simulink library "m3_common_lib"  (R2021b)
settings: Solver=ode45  StartTime=0.0  StopTime=10.0  RelTol=1e-3
undefined symbols (not defined in the file or in its folder): ACCEL_PRE_MULT, APDT_SrvcMgr_IRVHVDCSubFcnReq, C_C1GearNumbers, C_C1GearRatios, C_Calibration, C_DitherWaveform, C_GearOffset, C_GearRatioIn, C_GearRatioInverseOut, C_GearRatioOut, CLUTCH_INNER_LOOP_UPDATE_RATE, CONSTANT, DEGRADED_MODE_SIZE, Dem_EventStatusType, DiscIntNeverNeededParam, F_FAULT_ENUM, F_NOFAULT, F_OUTOFRANGE, F_RATELIMIT, FALSE, FMI14_SPECIAL_INSTRUCTIONS, FMI20_DATA_DRIFTED_HIGH, FMI21_DATA_DRIFTED_LOW, FMI29_RESERVED_FOR_SAE_ASSIGNMENT, FMI30_RESERVED_FOR_SAE_ASSIGNMENT, FMI31_CONDITION_EXISTS, FMI32_NO_FAULT, IC, k_accel, k_mean, MAX_UINT32, MEAN_PRE_MULT, NTriggers, QLTY_SIGNAL_FAILED, QLTY_SIGNAL_FULLY_FUNCTION, QLTY_SIGNAL_SUBSTITUTED_BY_1ST_CHOICE, QLTY_SIGNAL_SUBSTITUTED_BY_2ND_CHOICE, QLTY_SIGNAL_SUBSTITUTED_BY_3RD_CHOICE, QLTY_SIGNAL_SUBSTITUTED_BY_4TH_CHOICE, SAMPLE_TIME_100us, simin, T_TestPoint, TF_FALSE, TF_TRUE, TimeStep, TRUE, WORKSPACE_UPDATE_RATE, Zero, ZERO
libraries: $bdroot x121, simulink x23, simulink_extras x4, MBD_EPS_Local_Blockset x4
(part 5 of 10)

== system m3_common_lib/Diag/Fault Injection ==
  note: Common Library::Diagnostics::Fault Injection
  input : Inport
  gain : Inport  Port=2
  offset : Inport  Port=3
  ulim : Inport  Port=4
  llim : Inport  Port=5
  hold : Inport  Port=6
  fl_trigger : Inport  Port=7
  Gain and Offset (in) : $bdroot/SCond/Gain and Offset (in)  DataType=Double
  OOR Fault Detection : $bdroot/Diag/OOR Fault Detection  InitialValue=InitialValue
  Switch : Switch  Threshold=0.5  ZeroCross=off
  Unit Delay : UnitDelay  InitialCondition=InitialValue  SampleTime=-1  HasFrameUpgradeWarning=on
  output : Outport  VectorParamsAs1DForOutWhenUnconnected=off
  hwfl : Outport  Port=2  VectorParamsAs1DForOutWhenUnconnected=off
  wires:
  Gain and Offset (in)/1 -> Switch/3
  Switch/1 -> OOR Fault Detection/1
  Unit Delay/1 -> Switch/1
  hold/1 -> Switch/2
  llim/1 -> OOR Fault Detection/3
  ulim/1 -> OOR Fault Detection/2
  fl_trigger/1 -> OOR Fault Detection/4
  OOR Fault Detection/2 -> hwfl/1
  OOR Fault Detection/1 -> Unit Delay/1, output/1
  offset/1 -> Gain and Offset (in)/3
  gain/1 -> Gain and Offset (in)/2
  input/1 -> Gain and Offset (in)/1

== system m3_common_lib/Diag/Fault Log ==
  note: Common Library::Diagnostics::Fault Log
  HWfl_Active : Inport  OutDataTypeStr=boolean
  HWfl_Events : Inport  Port=2  OutDataTypeStr=uint16
  HWfl_Frames : Inport  Port=3  OutDataTypeStr=uint32
  hold : Inport  Port=4  OutDataTypeStr=boolean
  Constant1 : Constant  Value=EVENT_ZERO
  Constant18 : Constant  Value=EVENT_MAX
  Constant2 : Constant  Value=EVENT_ONE
  Constant3 : Constant  Value=FRAME_ZERO
  Constant4 : Constant  Value=FRAME_MAX
  Constant5 : Constant  Value=FRAME_ONE
  Logical Operator1 : Logic
  Logical Operator3 : Logic
  Logical Operator8 : Logic
  Sat : $bdroot/Slink/Sat
  Sat1 : $bdroot/Slink/Sat
  Sum : Sum  Inputs=|++  InputSameDT=on  OutDataTypeStr=Inherit: Same as first input
  Sum1 : Sum  Inputs=|++  InputSameDT=on  OutDataTypeStr=Inherit: Same as first input
  Unit Delay1 : UnitDelay  InitialCondition=false  SampleTime=-1  HasFrameUpgradeWarning=on
  not1 : Logic  Operator=NOT
  not2 : Logic  Operator=NOT
  reset switch : Switch  Criteria=u2 ~= 0  Threshold=0.5  ZeroCross=off  InputSameDT=on
  reset switch1 : Switch  Criteria=u2 ~= 0  Threshold=0.5  ZeroCross=off  InputSameDT=on
  events : Outport  VectorParamsAs1DForOutWhenUnconnected=off
  frames : Outport  Port=2  VectorParamsAs1DForOutWhenUnconnected=off
  wires:
  Logical Operator3/1 -> reset switch/2
  Logical Operator8/1 -> not1/1, Logical Operator3/1
  Unit Delay1/1 -> Logical Operator3/2
  not1/1 -> Unit Delay1/1
  Logical Operator1/1 -> reset switch1/2
  hold/1 -> not2/1
  not2/1 -> Logical Operator8/2, Logical Operator1/1
  HWfl_Frames/1 -> Sum1/2, reset switch1/3
  HWfl_Events/1 -> Sum/2, reset switch/3
  Constant5/1 -> Sum1/1
  Sat1/1 -> frames/1
  Sum1/1 -> reset switch1/1
  reset switch1/1 -> Sat1/1
  Constant3/1 -> Sat1/3
  Constant4/1 -> Sat1/2
  Constant2/1 -> Sum/1
  Sat/1 -> events/1
  Sum/1 -> reset switch/1
  reset switch/1 -> Sat/1
  Constant1/1 -> Sat/3
  Constant18/1 -> Sat/2
  HWfl_Active/1 -> Logical Operator1/2, Logical Operator8/1

== system m3_common_lib/Diag/Fault_Cntr ==
  note: Common Library::Diagnostics::Fault Counter
  fl : Inport  OutDataTypeStr=boolean
  reset : Inport  Port=2  OutDataTypeStr=boolean
  fmi : Inport  Port=3  OutDataTypeStr=uint16
  Constant1 : Constant  Value=up_cnt
  Constant10 : Constant  Value=red_light  OutDataTypeStr=boolean
  Constant2 : Constant  Value=dn_cnt
  Constant3 : Constant  Value=fc_level  OutDataTypeStr=int16
  Constant4 : Constant  Value=fault_id  OutDataTypeStr=uint16
  Constant6 : Constant  Value=amber_light  OutDataTypeStr=boolean
  Data Type Conversion : DataTypeConversion  OutDataTypeStr=uint16
  Data Type Conversion1 : DataTypeConversion  OutDataTypeStr=boolean
  Data Type Conversion2 : DataTypeConversion  OutDataTypeStr=int16
  Data Type Conversion3 : DataTypeConversion  OutDataTypeStr=int16
  FaultHandlerCoreLogic : Subsystem  TreatAsAtomicUnit=on  RTWFcnName=FC_FMI_Handler
      settings: RTWFcnNameOpts=User specified  RTWFileNameOpts=Use function name
  Signal Conversion : SignalConversion  ConversionOutput=Contiguous copy  OverrideOpt=on
  Signal Conversion1 : SignalConversion  ConversionOutput=Contiguous copy  OverrideOpt=on
  inc switch : Switch  Criteria=u2 ~= 0  Threshold=0.5  ZeroCross=off  InputSameDT=on
  fc : Outport  OutDataTypeStr=uint16  VectorParamsAs1DForOutWhenUnconnected=off
  lights : Outport  Port=2  OutDataTypeStr=uint8  VectorParamsAs1DForOutWhenUnconnected=off
  wires:
  fl/1 -> inc switch/2
  reset/1 -> Data Type Conversion1/1
  FaultHandlerCoreLogic/1(fc) -> Signal Conversion/1
  fmi/1 -> Data Type Conversion/1
  FaultHandlerCoreLogic/2(lights) -> Signal Conversion1/1
  Signal Conversion/1 -> fc/1
  Signal Conversion1/1 -> lights/1
  Data Type Conversion/1 -> FaultHandlerCoreLogic/3(fmi)
  Data Type Conversion1/1 -> FaultHandlerCoreLogic/2(reset)
  Constant2/1 -> inc switch/3
  Constant3/1 -> Data Type Conversion3/1
  Constant4/1 -> FaultHandlerCoreLogic/5(fid)
  Constant10/1 -> FaultHandlerCoreLogic/6(red)
  Constant6/1 -> FaultHandlerCoreLogic/7(amber)
  Constant1/1 -> inc switch/1
  inc switch/1 -> Data Type Conversion2/1
  Data Type Conversion2/1 -> FaultHandlerCoreLogic/1(fl)
  Data Type Conversion3/1 -> FaultHandlerCoreLogic/4(fc_level)

== system m3_common_lib/Diag/Filter w Fault Handler ==
  input : Inport
  tau : Inport  Port=2
  override_value : Inport  Port=3
  override? : Inport  Port=4
  reset? : Inport  Port=5
  default : Inport  Port=6
  ramp_time : Inport  Port=7
  fault? : Inport  Port=8
  Data Type Conversion{,1..4} (5 alike) : DataTypeConversion  OutDataTypeStr=single
  Data Type Conversion5 : DataTypeConversion  OutDataTypeStr=boolean
  Data Type Conversion6 : DataTypeConversion  OutDataTypeStr=boolean
  Data Type Conversion7 : DataTypeConversion  OutDataTypeStr=boolean
  FilterWithFaultHandlerCoreLogic : Subsystem  TreatAsAtomicUnit=on  RTWFcnName=FLTRWROFH
      settings: RTWFcnNameOpts=User specified  RTWFileNameOpts=Use function name
  Signal Conversion : SignalConversion  ConversionOutput=Contiguous copy  OverrideOpt=on
  output : Outport  VectorParamsAs1DForOutWhenUnconnected=off
  wires:
  input/1 -> Data Type Conversion/1
  tau/1 -> Data Type Conversion1/1
  override_value/1 -> Data Type Conversion2/1
  FilterWithFaultHandlerCoreLogic/1(output) -> Signal Conversion/1
  override?/1 -> Data Type Conversion7/1
  reset?/1 -> Data Type Conversion6/1
  default/1 -> Data Type Conversion3/1
  ramp_time/1 -> Data Type Conversion4/1
  fault?/1 -> Data Type Conversion5/1
  Signal Conversion/1 -> output/1
  Data Type Conversion/1 -> FilterWithFaultHandlerCoreLogic/1(input)
  Data Type Conversion1/1 -> FilterWithFaultHandlerCoreLogic/2(tau)
  Data Type Conversion2/1 -> FilterWithFaultHandlerCoreLogic/3(override_value)
  Data Type Conversion3/1 -> FilterWithFaultHandlerCoreLogic/6(default)
  Data Type Conversion4/1 -> FilterWithFaultHandlerCoreLogic/7(ramp_time)
  Data Type Conversion5/1 -> FilterWithFaultHandlerCoreLogic/8(fault?)
  Data Type Conversion6/1 -> FilterWithFaultHandlerCoreLogic/5(reset?)
  Data Type Conversion7/1 -> FilterWithFaultHandlerCoreLogic/4(override?)

== system m3_common_lib/Diag/Filter w Fault Handler1 ==
  note: Common Library::Diagnostics::Filter With Fault Handler
  input : Inport
  tau : Inport  Port=2
  reset? : Inport  Port=3
  default : Inport  Port=4
  ramp_time : Inport  Port=5
  fault? : Inport  Port=6
  Abs1 : Abs  ZeroCross=off
  Abs2 : Abs  ZeroCross=off
  Constant5 : Constant  Value=TimeStep
  Fltr_wRO : Subsystem  RTWFcnName=FLTRWRO  mask(CL Filter wRO){TimeStep=TimeStep}
      mask prompts: TimeStep "Time Step"
      mask help:
      | First Order Filter, y(n)= T/tau x(n) + (1 - T/tau) y(n-1)
      |
      | If override is true (1) then output=override_value
      | If      reset is true (1) then output=input
      |    otherwise output = previous output + (input - previous output) * T/tau
      |
      | X(1) = input
      | X(2) = tau
      | X(3) = override value
      | X(4) = override flag
      | X(5) = reset flag
      |
      | Y(1) = output
      |
      | Time step is entered via mask parameter.
      | NgEK, Inc.
      mask init:
      | switch class(TimeStep)
      |  case ('double')
      |       IC = double(0.0);
      |     case ('single')
      |        IC = single(0.0);
      |     case ('int8')
      |          IC = int8(0);
      |     case ('int16')
      |       IC = int16(0);
      |    case ('int32')
      |         IC = int32(0);
      | end;
      settings: RTWFileNameOpts=Use function name
      mask Help: web(which(['common_lib17.html']))
      mask Display:
      | patch([0.4 0.4 0.6 0.6], [0.35 0.65 0.65 0.35], [255/255 127/255 255/255])
      | disp('Filter\nw RO')
      | port_label('input', 1, 'input')
      | port_label('input', 2, 'tau')
      | port_label('input', 3, 'override_value')
      | port_label('input', 4, 'override?')
      | port_label('input', 5, 'reset?')
      | port_label('output', 1, 'output')
  Product1 : Product  Inputs=**/  InputSameDT=on  OutDataTypeStr=Inherit: Same as first input
  Sum1 : Sum  Inputs=+-|  InputSameDT=on  OutDataTypeStr=Inherit: Same as first input
  Sum2 : Sum  Inputs=+-|  InputSameDT=on  OutDataTypeStr=Inherit: Same as first input
  Sum3 : Sum  Inputs=+-|  InputSameDT=on  OutDataTypeStr=Inherit: Same as first input
  Switch{1..4} (4 alike) : Switch  Threshold=0.5  ZeroCross=off  InputSameDT=on
  delay : UnitDelay  InitialCondition=Zero  SampleTime=-1  HasFrameUpgradeWarning=on
  ic: signal at fault : UnitDelay  InitialCondition=Zero  SampleTime=-1  HasFrameUpgradeWarning=on
  within zero tol of corrections : RelationalOperator  Operator=<  ZeroCross=off  RndMeth=Nearest
  output : Outport  VectorParamsAs1DForOutWhenUnconnected=off
  wires:
  Sum3/1 -> Abs1/1
  delay/1 -> Switch2/1
  Switch3/1 -> delay/1
  within zero tol of corrections/1 -> Switch3/2
  Abs2/1 -> within zero tol of corrections/1
  Abs1/1 -> within zero tol of corrections/2
  Sum2/1 -> Switch3/1
  Switch1/1 -> Sum3/1, Sum2/1
  Switch4/1 -> Switch1/3, Sum1/1, ic: signal at fault/1
  ic: signal at fault/1 -> Switch4/1
  Product1/1 -> Abs2/1, Sum2/2
  Constant5/1 -> Product1/2
  Sum1/1 -> Product1/1
  default/1 -> Sum3/2, Switch3/3, Sum1/2
  Fltr_wRO/1(output) -> Switch4/3, output/1
  input/1 -> Switch2/3
  Switch2/1 -> Switch1/1, Fltr_wRO/1(input)
  reset?/1 -> Fltr_wRO/3(reset?)
  tau/1 -> Fltr_wRO/2(tau)
  fault?/1 -> Switch1/2, Switch4/2, Switch2/2
  ramp_time/1 -> Product1/3

== system m3_common_lib/Diag/OOR Fault Detection ==
  note: Common Library::Diagnostics::Out of Range Fault Detection
  in : Inport
  ulim : Inport  Port=2
  llim : Inport  Port=3
  ext_fault? : Inport  Port=4
  Logical Operator : Logic  Operator=OR  Inputs=3  AllPortsSameDT=off
  Relational Operator : RelationalOperator  Operator=<  ZeroCross=off  RndMeth=Nearest
  Relational Operator1 : RelationalOperator  Operator=<  ZeroCross=off  RndMeth=Nearest
  Sat : $bdroot/Slink/Sat
  Switch : Switch  Threshold=0.5  ZeroCross=off
  Unit Delay : UnitDelay  InitialCondition=InitialValue  SampleTime=-1  HasFrameUpgradeWarning=on
  out : Outport  VectorParamsAs1DForOutWhenUnconnected=off
  fault? : Outport  Port=2  VectorParamsAs1DForOutWhenUnconnected=off
  wires:
  Sat/1 -> Unit Delay/1, out/1
  Switch/1 -> Sat/1
  ext_fault?/1 -> Logical Operator/3
  llim/1 -> Sat/3, Relational Operator/2
  ulim/1 -> Relational Operator1/1, Sat/2
  in/1 -> Relational Operator1/2, Relational Operator/1, Switch/3
  Relational Operator1/1 -> Logical Operator/1
  Relational Operator/1 -> Logical Operator/2
  Logical Operator/1 -> Switch/2, fault?/1
  Unit Delay/1 -> Switch/1

== system m3_common_lib/Diag/Rate Limit Fault Detection ==
  note: Common Library::Diagnostics::Rate Limit Fault Detection
  in : Inport
  rlim : Inport  Port=2
  ext_fault? : Inport  Port=3
  Constant1 : Constant  Value=true
  Constant2 : Constant  Value=TimeStep
  Data Type Conversion : DataTypeConversion  OutDataTypeStr=single
  OOR Fault Detection : $bdroot/Diag/OOR Fault Detection  InitialValue=IC
  Product1 : Product  InputSameDT=on  OutDataTypeStr=Inherit: Same as first input
  Sum1 : Sum  Inputs=-+|  InputSameDT=on  OutDataTypeStr=Inherit: Same as first input
  Sum2 : Sum  Inputs=|++  InputSameDT=on  OutDataTypeStr=Inherit: Same as first input
  Sum3 : Sum  Inputs=++|  InputSameDT=on  OutDataTypeStr=Inherit: Same as first input
  Unit Delay : UnitDelay  InitialCondition=Zero  SampleTime=-1  HasFrameUpgradeWarning=on
      settings: AttributesFormatString=ic=%<X0>
  Unit Delay1 : UnitDelay  InitialCondition=false  SampleTime=-1  HasFrameUpgradeWarning=on
      settings: AttributesFormatString=ic=%<X0>
  Unit Delay2 : UnitDelay  InitialCondition=Zero  SampleTime=-1  HasFrameUpgradeWarning=on
      settings: AttributesFormatString=ic=%<X0>
  Unit Delay3 : UnitDelay  InitialCondition=false  SampleTime=-1  HasFrameUpgradeWarning=on
      settings: AttributesFormatString=ic=%<X0>
  inc switch : Switch  Threshold=0.5  ZeroCross=off  InputSameDT=on
  inc switch1 : Switch  Threshold=0.5  ZeroCross=off  InputSameDT=on
  out : Outport  VectorParamsAs1DForOutWhenUnconnected=off
  fault? : Outport  Port=2  VectorParamsAs1DForOutWhenUnconnected=off
  wires:
  Constant2/1 -> Data Type Conversion/1
  Data Type Conversion/1 -> Product1/1
  inc switch1/1 -> Sum2/1, Sum1/2
  Unit Delay3/1 -> inc switch1/2
  Constant1/1 -> Unit Delay3/1
  Unit Delay/1 -> inc switch1/1
  Unit Delay1/1 -> inc switch/2
  Unit Delay2/1 -> Sum3/1
  Sum3/1 -> inc switch/1
  Product1/1 -> Sum3/2, inc switch/3
  rlim/1 -> Product1/2
  inc switch/1 -> Unit Delay2/1, Sum1/1, Sum2/2
  Sum2/1 -> OOR Fault Detection/2
  Sum1/1 -> OOR Fault Detection/3
  OOR Fault Detection/2 -> Unit Delay1/1, fault?/1
  OOR Fault Detection/1 -> Unit Delay/1, out/1
  ext_fault?/1 -> OOR Fault Detection/4
  in/1 -> inc switch1/3, OOR Fault Detection/1

== system m3_common_lib/Diagnostics/Calibration Enabled Debounce ==
  diagInput : Inport
  diagStartUpComp : Inport  Port=2
  diagMaxVal : Inport  Port=3
  diagMinVal : Inport  Port=4
  diagUpCnt : Inport  Port=5
  diagDnCnt : Inport  Port=6
  diagFaultCntThresh : Inport  Port=7
  diagPassCntThresh : Inport  Port=8
  diagDbncEnab : Inport  Port=9
  diagReset : Inport  Port=10
  diagEnable : Inport  Port=11
  diagHealEn : Inport  Port=12
  DiagFaultCounter : $bdroot/Diagnostics/DiagFaultCounter  SystemSampleTime=-1  VariantActivationTime=update diagram  Latency=0  AutoFrameSizeCalculation=off
  OR : Logic  Operator=OR  AllPortsSameDT=off  OutDataTypeStr=boolean
  Relational Operator : RelationalOperator  OutDataTypeStr=boolean  ZeroCross=off  RndMeth=Nearest
  Relational Operator1 : RelationalOperator  Operator=<=  OutDataTypeStr=boolean  ZeroCross=off  RndMeth=Nearest
  diagFaultStatus : Outport  OutputWhenDisabled=reset  InitialOutput=Dem_EventStatusType.DEM_EVENT_STATUS_INIT  VectorParamsAs1DForOutWhenUnconnected=off
  wires:
  diagHealEn/1 -> DiagFaultCounter/10
  diagPassCntThresh/1 -> DiagFaultCounter/7
  diagMaxVal/1 -> Relational Operator/2
  diagMinVal/1 -> Relational Operator1/2
  Relational Operator/1 -> OR/1
  Relational Operator1/1 -> OR/2
  diagInput/1 -> Relational Operator/1, Relational Operator1/1
  OR/1 -> DiagFaultCounter/1
  diagStartUpComp/1 -> DiagFaultCounter/2
  diagReset/1 -> DiagFaultCounter/3
  diagEnable/1 -> DiagFaultCounter/4
  diagDbncEnab/1 -> DiagFaultCounter/5
  diagFaultCntThresh/1 -> DiagFaultCounter/6
  diagUpCnt/1 -> DiagFaultCounter/8
  diagDnCnt/1 -> DiagFaultCounter/9
  DiagFaultCounter/1 -> diagFaultStatus/1

== system m3_common_lib/Diagnostics/Calibration Enabled Debounce Boolean Input ==
  diagInput : Inport
  diagStartUpComp : Inport  Port=2
  diagUpCnt : Inport  Port=3
  diagDnCnt : Inport  Port=4
  diagFaultCntThresh : Inport  Port=5
  diagPassCntThresh : Inport  Port=6
  diagDbncEnab : Inport  Port=7
  diagReset : Inport  Port=8
  diagEnable : Inport  Port=9
  diagHealEn : Inport  Port=10
  DiagFaultCounter : $bdroot/Diagnostics/DiagFaultCounter  SystemSampleTime=-1  VariantActivationTime=update diagram  Latency=0  AutoFrameSizeCalculation=off
  diagFaultStatus : Outport  OutputWhenDisabled=reset  InitialOutput=Dem_EventStatusType.DEM_EVENT_STATUS_INIT  VectorParamsAs1DForOutWhenUnconnected=off
  wires:
  DiagFaultCounter/1 -> diagFaultStatus/1
  diagDnCnt/1 -> DiagFaultCounter/9
  diagUpCnt/1 -> DiagFaultCounter/8
  diagFaultCntThresh/1 -> DiagFaultCounter/6
  diagDbncEnab/1 -> DiagFaultCounter/5
  diagEnable/1 -> DiagFaultCounter/4
  diagReset/1 -> DiagFaultCounter/3
  diagStartUpComp/1 -> DiagFaultCounter/2
  diagInput/1 -> DiagFaultCounter/1
  diagPassCntThresh/1 -> DiagFaultCounter/7
  diagHealEn/1 -> DiagFaultCounter/10

== system m3_common_lib/Diagnostics/Calibration Enabled MinMax OOR ==
  Input : Inport
  ULim : Inport  Port=2
  LLim : Inport  Port=3
  Cal_Enable : Inport  Port=4
  Ext_Fault : Inport  Port=5
  Enabled OOR : Subsystem  mask(Enabled OOR Subsystem){InitialValue=InitialValue, InDataType=single}
      mask prompts: InitialValue "Initial Value"; InDataType "Input Data Type"
      mask init:
      | DataType = get_param(gcb, 'InDataType');
      | Capture1 = [gcb '/OOR MinMax Capture/CL MinMax Capture'];
      | Capture2 = [gcb '/OOR MinMax Capture/CL MinMax Capture1'];
      | 
      | set_param(Capture1, 'InDataType', DataType);
      | set_param(Capture2, 'InDataType', DataType);
      mask TypeOptions InDataType: single | int16
  Switch : Switch  Threshold=0.5  ZeroCross=off
  Switch1 : Switch  Threshold=0.5  ZeroCross=off
  Out : Outport  VectorParamsAs1DForOutWhenUnconnected=off
  Max_Value : Outport  Port=2  VectorParamsAs1DForOutWhenUnconnected=off
  Min_Value : Outport  Port=3  VectorParamsAs1DForOutWhenUnconnected=off
  Fault : Outport  Port=4  VectorParamsAs1DForOutWhenUnconnected=off
  wires:
  Input/1 -> Enabled OOR/1(In), Switch/3
  ULim/1 -> Enabled OOR/2(ULim)
  LLim/1 -> Enabled OOR/3(LLim)
  Ext_Fault/1 -> Enabled OOR/4(Ext_Fault), Switch1/3
  Switch/1 -> Out/1
  Switch1/1 -> Fault/1
  Enabled OOR/1(Out) -> Switch/1
  Cal_Enable/1 -> Switch1/2, Switch/2, Enabled OOR/Enable
  Enabled OOR/2(Fault) -> Switch1/1
  Enabled OOR/3(Max) -> Max_Value/1
  Enabled OOR/4(Min) -> Min_Value/1

== system m3_common_lib/Diagnostics/Calibration Enabled MinMax RLim ==
  Input : Inport
  Rate_Limit : Inport  Port=2
  Cal_Enable : Inport  Port=3
  Ext_Fault : Inport  Port=4
  Enabled RLim : Subsystem  mask(Enablede Rate Limit Fault Detection){IC=IC, TimeStep=TimeStep, InDataType=single}
      mask prompts: IC "Initial Condition"; TimeStep "Update Time"; InDataType "Input Data Type"
      mask init:
      | DataType = get_param(gcb, 'InDataType');
      | Capture1 = [gcb '/RLim MinMax Capture/CL MinMax Capture'];
      | Capture2 = [gcb '/RLim MinMax Capture/CL MinMax Capture1'];
      | 
      | set_param(Capture1, 'InDataType', DataType);
      | set_param(Capture2, 'InDataType', DataType);
      mask TypeOptions InDataType: single | int16
  Switch : Switch  Threshold=0.5  ZeroCross=off
  Switch1 : Switch  Threshold=0.5  ZeroCross=off
  Out : Outport  VectorParamsAs1DForOutWhenUnconnected=off
  Max Pos Rate : Outport  Port=2  VectorParamsAs1DForOutWhenUnconnected=off
  Max Neg Rate : Outport  Port=3  VectorParamsAs1DForOutWhenUnconnected=off
  Fault : Outport  Port=4  VectorParamsAs1DForOutWhenUnconnected=off
  wires:
  Cal_Enable/1 -> Switch/2, Switch1/2, Enabled RLim/Enable
  Input/1 -> Switch/3, Enabled RLim/1(In)
  Switch/1 -> Out/1
  Switch1/1 -> Fault/1
  Rate_Limit/1 -> Enabled RLim/2(RLim)
  Enabled RLim/1(out) -> Switch/1
  Enabled RLim/2(fault?) -> Switch1/1
  Ext_Fault/1 -> Enabled RLim/3(Ext_Fault), Switch1/3
  Enabled RLim/3(Max Pos Rate) -> Max Pos Rate/1
  Enabled RLim/4(Max Neg Rate) -> Max Neg Rate/1

== system m3_common_lib/Diagnostics/Ccaller_DiagLv1 ==
  diagFaultActive : Inport
  diagStartUpComp : Inport  Port=2
  diagReset : Inport  Port=3
  diagEnable : Inport  Port=4
  diagDbncEnable : Inport  Port=5
  diagFaultCntThresh : Inport  Port=6
  diagPassCntThresh : Inport  Port=7
  diagUpCnt : Inport  Port=8
  diagDnCnt : Inport  Port=9
  diagHealEn : Inport  Port=10
  diagPrestorageEn : Inport  Port=11
  diagJumpDownEn : Inport  Port=12
  DiagDebounceLv1_CCaller : CCaller  FunctionName=DiagDebounceLv1  PortSpecificationStruct="%)30     .    <!<   8    (     @         %    \"     T    !     0         %  0 \"0    $    _    07)G3F%M90  4&]R=$YA;64 4V-O<&4     26YD97@     5'EP90      4VEZ90      27-';&]B86P   X   !     !@    @    $          4    (     0   !     !         !     0    9&EA9T9A=6QT0V]U;G1E<@X   !     !@    @    $          4    (     0   !     !         !     0    9&EA9T9A=6QT0V]U;G1E<@X   !     !@    @    $     ...(+7711 chars)"
  Unit Delay : UnitDelay  InitialCondition=int16(0)  SampleTime=-1  HasFrameUpgradeWarning=on
      settings: AttributesFormatString=%<InitialCondition>
  Unit Delay1 : UnitDelay  InitialCondition=uint8(32)  SampleTime=-1  HasFrameUpgradeWarning=on
      settings: AttributesFormatString=%<InitialCondition>
  Unit Delay2 : UnitDelay  InitialCondition=false  SampleTime=-1  HasFrameUpgradeWarning=on
      settings: AttributesFormatString=%<InitialCondition>
  Unit Delay3 : UnitDelay  InitialCondition=false  SampleTime=-1  HasFrameUpgradeWarning=on
      settings: AttributesFormatString=%<InitialCondition>
  Unit Delay4 : UnitDelay  InitialCondition=false  SampleTime=-1  HasFrameUpgradeWarning=on
      settings: AttributesFormatString=%<InitialCondition>
  diagFaultStatus : Outport  VectorParamsAs1DForOutWhenUnconnected=off
  diagPrestorageTrigger : Outport  Port=2  VectorParamsAs1DForOutWhenUnconnected=off
  wires:
  diagJumpDownEn/1 -> ?
  Unit Delay4/1 -> DiagDebounceLv1_CCaller/4
  ? -> Unit Delay4/1
  diagPrestorageEn/1 -> ?
  Unit Delay3/1 -> DiagDebounceLv1_CCaller/5
  ? -> diagPrestorageTrigger/1, Unit Delay3/1
  Unit Delay2/1 -> DiagDebounceLv1_CCaller/3
  DiagDebounceLv1_CCaller/3 -> Unit Delay2/1
  Unit Delay1/1 -> DiagDebounceLv1_CCaller/2
  DiagDebounceLv1_CCaller/2 -> Unit Delay1/1, diagFaultStatus/1
  Unit Delay/1 -> DiagDebounceLv1_CCaller/1
  DiagDebounceLv1_CCaller/1 -> Unit Delay/1
  diagPassCntThresh/1 -> DiagDebounceLv1_CCaller/12
  diagDbncEnable/1 -> DiagDebounceLv1_CCaller/10
  diagEnable/1 -> DiagDebounceLv1_CCaller/9
  diagHealEn/1 -> ?
  diagFaultActive/1 -> DiagDebounceLv1_CCaller/6
  diagFaultCntThresh/1 -> DiagDebounceLv1_CCaller/11
  diagReset/1 -> DiagDebounceLv1_CCaller/8
  diagDnCnt/1 -> ?
  diagStartUpComp/1 -> DiagDebounceLv1_CCaller/7
  diagUpCnt/1 -> DiagDebounceLv1_CCaller/13

== system m3_common_lib/Diagnostics/Ccaller_DiagLv2 ==
  diagFaultActive : Inport
  diagStartUpComp : Inport  Port=2
  diagReset : Inport  Port=3
  diagFaultCntThresh : Inport  Port=4
  diagUpCnt : Inport  Port=5
  diagDnCnt : Inport  Port=6
  diagHealEn : Inport  Port=7
  DiagDebounceLv2_CCaller : CCaller  FunctionName=DiagDebounceLv2  PortSpecificationStruct="%)30     .    8!$   8    (     @         %    \"     L    !     0         %  0 \"0    $    V    07)G3F%M90  4&]R=$YA;64 4V-O<&4     26YD97@     5'EP90      4VEZ90         .    ,     8    (    !          %    \"     $    #     0         0  , ;W5T  X    P    !@    @    $          4    (     0    ,    !         !   P!O=70 #@   #@    &    \"     0         !0    @    !    !@    $         $     8   !/=7 ...(+5614 chars)"
  Unit Delay : UnitDelay  InitialCondition=int16(0)  SampleTime=-1  HasFrameUpgradeWarning=on
      settings: AttributesFormatString=%<InitialCondition>
  Unit Delay1 : UnitDelay  InitialCondition=uint8(0)  SampleTime=-1  HasFrameUpgradeWarning=on
      settings: AttributesFormatString=%<InitialCondition>
  Unit Delay2 : UnitDelay  InitialCondition=int16(0)  SampleTime=-1  HasFrameUpgradeWarning=on
      settings: AttributesFormatString=%<InitialCondition>
  diagFaultStatus : Outport  VectorParamsAs1DForOutWhenUnconnected=off
  wires:
  diagUpCnt/1 -> DiagDebounceLv2_CCaller/8
  diagStartUpComp/1 -> DiagDebounceLv2_CCaller/5
  diagDnCnt/1 -> DiagDebounceLv2_CCaller/9
  diagReset/1 -> DiagDebounceLv2_CCaller/6
  DiagDebounceLv2_CCaller/1 -> diagFaultStatus/1
  diagFaultCntThresh/1 -> DiagDebounceLv2_CCaller/7
  diagFaultActive/1 -> DiagDebounceLv2_CCaller/4
  diagHealEn/1 -> DiagDebounceLv2_CCaller/10
  DiagDebounceLv2_CCaller/2 -> Unit Delay/1
  Unit Delay/1 -> DiagDebounceLv2_CCaller/1
  DiagDebounceLv2_CCaller/3 -> Unit Delay1/1
  Unit Delay1/1 -> DiagDebounceLv2_CCaller/2
  DiagDebounceLv2_CCaller/4 -> Unit Delay2/1
  Unit Delay2/1 -> DiagDebounceLv2_CCaller/3

== system m3_common_lib/Diagnostics/DiagFaultCounter ==
  diagFaultActive : Inport
  diagStartUpComp : Inport  Port=2
  diagReset : Inport  Port=3
  diagEnable : Inport  Port=4
  diagDbncEnab : Inport  Port=5
  diagFaultCntThresh : Inport  Port=6
  diagPassCntThresh : Inport  Port=7
  diagUpCnt : Inport  Port=8
  diagDnCnt : Inport  Port=9
  diagHealEn : Inport  Port=10
  DiagFaulCounter : Stateflow chart  TreatAsAtomicUnit=on
  diagFaultStatus : Outport  OutputWhenDisabled=reset  InitialOutput=Dem_EventStatusType.DEM_EVENT_STATUS_INIT  VectorParamsAs1DForOutWhenUnconnected=off
  wires:
  diagHealEn/1 -> DiagFaulCounter/10(diagHealEn)
  diagPassCntThresh/1 -> DiagFaulCounter/7(diagPassCntThresh)
  diagStartUpComp/1 -> DiagFaulCounter/2(diagStartUpComp)
  diagDbncEnab/1 -> DiagFaulCounter/5(diagDbncEnab)
  DiagFaulCounter/1(diagFaultStatus) -> diagFaultStatus/1
  diagEnable/1 -> DiagFaulCounter/4(diagEnable)
  diagDnCnt/1 -> DiagFaulCounter/9(diagDnCnt)
  diagUpCnt/1 -> DiagFaulCounter/8(diagUpCnt)
  diagReset/1 -> DiagFaulCounter/3(diagReset)
  diagFaultCntThresh/1 -> DiagFaulCounter/6(diagFaultCntThresh)
  diagFaultActive/1 -> DiagFaulCounter/1(diagFaultActive)

== system m3_common_lib/Diagnostics/ExtractValue ==
  in : Inport  OutDataTypeStr=Bus: BO_InputSignal
  Bus Selector : BusSelector  OutputSignals=value,FMI
  value : Outport  VectorParamsAs1DForOutWhenUnconnected=off
  FMI : Outport  Port=2  VectorParamsAs1DForOutWhenUnconnected=off
  wires:
  Bus Selector/2 -> FMI/1  "<FMI>"
  in/1 -> Bus Selector/1
  Bus Selector/1 -> value/1  "<value>"

== system m3_common_lib/Diagnostics/FMIUpdate ==
  UpdateFaultStatus : Inport
  FMI_In : Inport  Port=2
  FMI_UpdateValue : Inport  Port=3
  Constant2 : Constant  Value=FMI32_NO_FAULT  SampleTime=-1
  Relational Operator3 : RelationalOperator  Operator=~=  ZeroCross=off  RndMeth=Nearest
  Switch : Switch  Threshold=0.5  ZeroCross=off
  Switch1 : Switch  Threshold=0.5  ZeroCross=off
  FMI_Out : Outport  VectorParamsAs1DForOutWhenUnconnected=off
  wires:
  Switch1/1 -> FMI_Out/1
  FMI_In/1 -> Switch/3, Switch1/1, Relational Operator3/1
  Relational Operator3/1 -> Switch1/2
  Switch/1 -> Switch1/3
  FMI_UpdateValue/1 -> Switch/1
  UpdateFaultStatus/1 -> Switch/2
  Constant2/1 -> Relational Operator3/2

== system m3_common_lib/Diagnostics/Fault Debounce Lv1 Boolean Input ==
  diagInput : Inport
  diagStartUpComp : Inport  Port=2
  diagUpCnt : Inport  Port=3
  diagDnCnt : Inport  Port=4
  diagFaultCntThresh : Inport  Port=5
  diagPassCntThresh : Inport  Port=6
  diagDbncEnab : Inport  Port=7
  diagReset : Inport  Port=8
  diagEnable : Inport  Port=9
  diagHealEn : Inport  Port=10
  diagPreestorageEn : Inport  Port=11
  diagJumpDownEn : Inport  Port=12
  Ccaller_DiagLv1 : $bdroot/Diagnostics/Ccaller_DiagLv1  SystemSampleTime=-1  VariantActivationTime=update diagram  Latency=0  AutoFrameSizeCalculation=off
  diagFaultStatus : Outport  OutputWhenDisabled=reset  InitialOutput=Dem_EventStatusType.DEM_EVENT_STATUS_INIT  VectorParamsAs1DForOutWhenUnconnected=off
  diagPreestorageTrigger : Outport  Port=2  OutputWhenDisabled=reset  InitialOutput=Dem_EventStatusType.DEM_EVENT_STATUS_INIT  VectorParamsAs1DForOutWhenUnconnected=off
  wires:
  diagStartUpComp/1 -> Ccaller_DiagLv1/2
  diagReset/1 -> Ccaller_DiagLv1/3
  diagEnable/1 -> Ccaller_DiagLv1/4
  diagDbncEnab/1 -> Ccaller_DiagLv1/5
  diagFaultCntThresh/1 -> Ccaller_DiagLv1/6
  diagPassCntThresh/1 -> Ccaller_DiagLv1/7
  diagUpCnt/1 -> Ccaller_DiagLv1/8
  diagDnCnt/1 -> Ccaller_DiagLv1/9
  diagHealEn/1 -> Ccaller_DiagLv1/10
  diagPreestorageEn/1 -> Ccaller_DiagLv1/11
  diagJumpDownEn/1 -> Ccaller_DiagLv1/12
  Ccaller_DiagLv1/2 -> diagPreestorageTrigger/1
  Ccaller_DiagLv1/1 -> diagFaultStatus/1
  diagInput/1 -> Ccaller_DiagLv1/1

== system m3_common_lib/Diagnostics/Fault Debounce Lv1 state Input ==
  diagInput : Inport
  diagStartUpComp : Inport  Port=2
  diagMaxVal : Inport  Port=3
  diagMinVal : Inport  Port=4
  diagUpCnt : Inport  Port=5
  diagDnCnt : Inport  Port=6
  diagFaultCntThresh : Inport  Port=7
  diagPassCntThresh : Inport  Port=8
  diagDbncEnab : Inport  Port=9
  diagReset : Inport  Port=10
  diagEnable : Inport  Port=11
  diagHealEn : Inport  Port=12
  diagPreestorageEn : Inport  Port=13
  diagJumpDownEn : Inport  Port=14
  Ccaller_DiagLv1 : $bdroot/Diagnostics/Ccaller_DiagLv1  SystemSampleTime=-1  VariantActivationTime=update diagram  Latency=0  AutoFrameSizeCalculation=off
  OR : Logic  Operator=OR  AllPortsSameDT=off  OutDataTypeStr=boolean
  Relational Operator : RelationalOperator  OutDataTypeStr=boolean  ZeroCross=off  RndMeth=Nearest
  Relational Operator1 : RelationalOperator  Operator=<=  OutDataTypeStr=boolean  ZeroCross=off  RndMeth=Nearest
  diagFaultStatus : Outport  OutputWhenDisabled=reset  InitialOutput=Dem_EventStatusType.DEM_EVENT_STATUS_INIT  VectorParamsAs1DForOutWhenUnconnected=off
  diagPreestorageTrigger : Outport  Port=2  OutputWhenDisabled=reset  InitialOutput=Dem_EventStatusType.DEM_EVENT_STATUS_INIT  VectorParamsAs1DForOutWhenUnconnected=off
  wires:
  diagMaxVal/1 -> Relational Operator/2
  diagReset/1 -> Ccaller_DiagLv1/3
  diagDnCnt/1 -> Ccaller_DiagLv1/9
  diagFaultCntThresh/1 -> Ccaller_DiagLv1/6
  diagPassCntThresh/1 -> Ccaller_DiagLv1/7
  diagUpCnt/1 -> Ccaller_DiagLv1/8
  Relational Operator/1 -> OR/1
  diagStartUpComp/1 -> Ccaller_DiagLv1/2
  diagDbncEnab/1 -> Ccaller_DiagLv1/5
  diagInput/1 -> Relational Operator/1, Relational Operator1/1
  diagHealEn/1 -> Ccaller_DiagLv1/10
  diagMinVal/1 -> Relational Operator1/2
  OR/1 -> Ccaller_DiagLv1/1
  Relational Operator1/1 -> OR/2
  diagEnable/1 -> Ccaller_DiagLv1/4
  diagPreestorageEn/1 -> Ccaller_DiagLv1/11
  diagJumpDownEn/1 -> Ccaller_DiagLv1/12
  Ccaller_DiagLv1/1 -> diagFaultStatus/1
  Ccaller_DiagLv1/2 -> diagPreestorageTrigger/1

== system m3_common_lib/Diagnostics/FaultStatusUpdate ==
  FMI_In : Inport
  DriftLow : Inport  Port=2
  DriftHigh : Inport  Port=3
  SpecialInstructions : Inport  Port=4
  ConditionExists : Inport  Port=5
  DriftLowSubReqest : Inport  Port=6
  DriftLowSubReqest1 : Inport  Port=7
  Constant : Constant  Value=FMI14_SPECIAL_INSTRUCTIONS  SampleTime=-1
  Constant1 : Constant  Value=FMI21_DATA_DRIFTED_LOW  SampleTime=-1
  Constant2 : Constant  Value=FMI20_DATA_DRIFTED_HIGH  SampleTime=-1
  Constant3 : Constant  Value=FMI29_RESERVED_FOR_SAE_ASSIGNMENT  SampleTime=-1
  Constant4 : Constant  Value=FMI32_NO_FAULT  SampleTime=-1
  Constant5 : Constant  Value=FMI30_RESERVED_FOR_SAE_ASSIGNMENT  SampleTime=-1
  Constant6 : Constant  Value=FMI31_CONDITION_EXISTS  SampleTime=-1
  Relational Operator3 : RelationalOperator  Operator=~=  ZeroCross=off  RndMeth=Nearest
  Switch{,1..6} (7 alike) : Switch  Threshold=0.5  ZeroCross=off
  FMI_Out : Outport  VectorParamsAs1DForOutWhenUnconnected=off
  wires:
  Switch1/1 -> FMI_Out/1
  Constant4/1 -> Relational Operator3/2
  Switch/1 -> Switch1/3
  Relational Operator3/1 -> Switch1/2
  FMI_In/1 -> Relational Operator3/1, Switch1/1, Switch6/3
  Switch2/1 -> Switch/3
  Switch3/1 -> Switch2/3
  Switch4/1 -> Switch3/3
  DriftLow/1 -> Switch/2
  Constant1/1 -> Switch/1
  Constant2/1 -> Switch2/1
  DriftHigh/1 -> Switch2/2
  Constant/1 -> Switch3/1
  SpecialInstructions/1 -> Switch3/2
  Constant6/1 -> Switch4/1
  ConditionExists/1 -> Switch4/2
  Constant3/1 -> Switch5/1
  DriftLowSubReqest/1 -> Switch5/2
  Constant5/1 -> Switch6/1
  DriftLowSubReqest1/1 -> Switch6/2
  Switch6/1 -> Switch5/3
  Switch5/1 -> Switch4/3

== system m3_common_lib/Diagnostics/KeepAlive ==
  State : Inport  OutDataTypeStr=boolean  PortDimensions=1
  A : Inport  Port=2  PortDimensions=1
  B : Inport  Port=3  PortDimensions=1
  Delay : UnitDelay  InitialCondition=false  SampleTime=-1  HasFrameUpgradeWarning=on
  Logical Operator : Logic  Operator=OR  AllPortsSameDT=off  OutDataTypeStr=boolean
  RelOp : RelationalOperator  Operator===  OutDataTypeStr=boolean  RndMeth=Nearest  InputSameDT=on
  Enable : Outport  OutDataTypeStr=boolean  PortDimensions=1  VectorParamsAs1DForOutWhenUnconnected=off
  Rel : Outport  Port=2  OutDataTypeStr=boolean  PortDimensions=1  VectorParamsAs1DForOutWhenUnconnected=off
  wires:
  RelOp/1 -> Logical Operator/2, Rel/1
  Logical Operator/1 -> Enable/1
  B/1 -> RelOp/2
  Delay/1 -> Logical Operator/1
  State/1 -> Delay/1
  A/1 -> RelOp/1

== system m3_common_lib/Diagnostics/LogicBasedActivation ==
  note: Logic Based Activation
  Enable : Inport  OutDataTypeStr=boolean  PortDimensions=1
  DMToAdd : Inport  Port=2  OutDataTypeStr=uint32  PortDimensions=DM_SIZE
  Add : Inport  Port=3  OutDataTypeStr=boolean  PortDimensions=1
  DMPackedData_in : Inport  Port=4  OutDataTypeStr=uint32  PortDimensions=DM_SIZE
  Bitwise Operator : simulink/Logic and Bit Operations/Bitwise Operator  logicop=OR  UseBitMask=off  NumInputPorts=2  BitMask=bin2dec('11011001')  BitMaskRealWorld=Stored Integer
  Logical Operator1 : Logic  AllPortsSameDT=off
  Switch3 : Switch  Threshold=0.5  ZeroCross=off
  DMPackedData_out : Outport  OutDataTypeStr=uint32  PortDimensions=DM_SIZE  VectorParamsAs1DForOutWhenUnconnected=off
  wires:
  Switch3/1 -> DMPackedData_out/1
  Bitwise Operator/1 -> Switch3/1
  DMToAdd/1 -> Bitwise Operator/1
  DMPackedData_in/1 -> Bitwise Operator/2, Switch3/3
  Logical Operator1/1 -> Switch3/2
  Enable/1 -> Logical Operator1/1
  Add/1 -> Logical Operator1/2

== system m3_common_lib/Diagnostics/LogicBasedDeactivation ==
  note: Logic Based Deactivation
  Enable : Inport  OutDataTypeStr=boolean  PortDimensions=1
  DMToRemove : Inport  Port=2  OutDataTypeStr=uint32  PortDimensions=DM_SIZE
  Remove : Inport  Port=3  OutDataTypeStr=boolean  PortDimensions=1
  DMPackedData_in : Inport  Port=4  OutDataTypeStr=uint32  PortDimensions=DM_SIZE
  Bitwise Operator : simulink/Logic and Bit Operations/Bitwise Operator  logicop=AND  UseBitMask=off  NumInputPorts=2  BitMask=bin2dec('11011001')  BitMaskRealWorld=Stored Integer
  Bitwise Operator1 : simulink/Logic and Bit Operations/Bitwise Operator  logicop=NOT  UseBitMask=off  BitMask=bin2dec('11011001')  BitMaskRealWorld=Stored Integer
  Logical Operator1 : Logic  AllPortsSameDT=off
  Switch3 : Switch  Threshold=0.5  ZeroCross=off
  DMPackedData_out : Outport  OutDataTypeStr=uint32  PortDimensions=DM_SIZE  VectorParamsAs1DForOutWhenUnconnected=off
  wires:
  Remove/1 -> Logical Operator1/2
  Enable/1 -> Logical Operator1/1
  Logical Operator1/1 -> Switch3/2
  DMPackedData_in/1 -> Switch3/3, Bitwise Operator/2
  DMToRemove/1 -> Bitwise Operator1/1
  Bitwise Operator/1 -> Switch3/1
  Switch3/1 -> DMPackedData_out/1
  Bitwise Operator1/1 -> Bitwise Operator/1
